simulink model "Geneerator"  (R2022b)
settings: Solver=VariableStepAuto  StartTime=0.0  StopTime=10.0  RelTol=1e-3
settings Model: Creator=mliu  LastModifiedBy=mliu

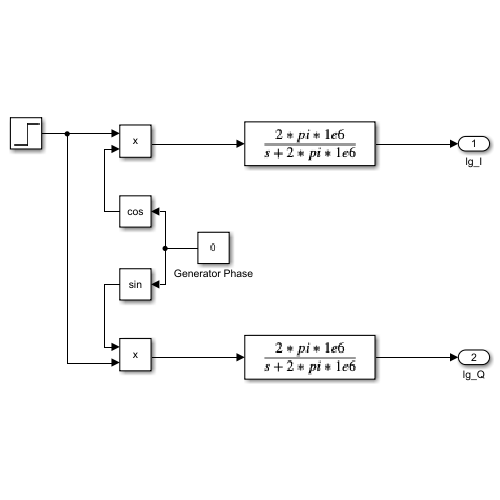
[thumbnail: Simulink's stored preview of the top-level diagram]
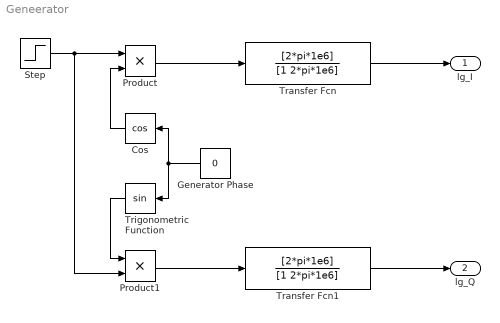
== system Geneerator ==
  Cos : Trigonometry  Operator=cos
  Generator Phase : Constant  Value=0
  Product : Product
  Product1 : Product
  Step : Step  SampleTime=0
  Transfer Fcn : TransferFcn  Numerator=[2*pi*1e6]  Denominator=[1 2*pi*1e6]
  Transfer Fcn1 : TransferFcn  Numerator=[2*pi*1e6]  Denominator=[1 2*pi*1e6]
  Trigonometric Function : Trigonometry
  lg_I : Outport
  lg_Q : Outport  Port=2
  wires:
  Step/1 -> Product1/2, Product/1
  Cos/1 -> Product/2
  Generator Phase/1 -> Trigonometric Function/1, Cos/1
  Trigonometric Function/1 -> Product1/1
  Product/1 -> Transfer Fcn/1
  Product1/1 -> Transfer Fcn1/1
  Transfer Fcn/1 -> lg_I/1
  Transfer Fcn1/1 -> lg_Q/1
